simulink model "EV_PV_Charging"  (R2025a)
settings: Solver=ode3  StartTime=0.0  StopTime=1  RelTol=1e-3
PreLoadFcn:
  | %% Parameter file: OBC_4_data.m
  | 
  | %% Model Parameters
  | Ts_Power= 50e-9;        % SPS Model sample time (s)
  | Co=150e-6;              % Output filter (F)
  | Ron_FET=50e-3;          % FET resistance (ohms)
  | Ron_Diode=50e-3;        % FET resistance (ohms)
  | Vf=0.6;                 % Diode forward voltage (V)
  | %
  | %% PFC Data
  | Vnom_ac= 240;           % Nominal Ac voltage (V)
  | Fnom= 60;               % System frequency (Hz)
  | L_PFC= 600e-6;          % PFC Inductance (H)
  | RL_PFC= 20e-3;          % Inductance resistance (Ohm)
  | C_PFC= 2600e-6;         % Capacitance (F)
  | 
  | %% PFC Control System Parameters
  | Ts_Control= 10e-6;      % Control system time (s)
  | Fsw= 100e3;             % PWM Switching frequency (Hz)
  | DT_PFC=400e-9;
  | %
  | % Current Regulator (PR):
  | Kp_I= 0.06;             % Proportional gain
  | Kr_I= 2.5;              % Resonant gain
  | Zeta_I=0.2;             % Damping coefficient
  | Fr_I=Fnom*2;            % Resonant frequency (Hz)
  | %
  | % Voltage Regulator (PI):
  | Kp_V= 0.25;             % Proportional gain
  | Ki_V= 80;               % Integral gain
  | Limit_V= 100;           % Output limit
  | %
  | %% LLC Data
  | Vdc_in=400;             % DC input voltage (V)
  | Vo_nom=400;             % DC nominal output voltage (V)
  | Po_nom=7.2e3;           % Nominal output power (W)
  | Lr=25e-6;               % Transformer leakage inductance (Resonant inductance in Henry)
  | Lm=150e-6;              % Magnetization inductance (H)
  | Cr=75e-9;               % Resonant capacitor (F)
  | Np=10; Ns=12; N=Np/Ns;  % Transformer ratio
  | %
  | %% LLC Control System Parameters
  | DT_LLC=400e-9;
  | Ts_Control=10e-6;
  | % Voltage Regulator (PI):
  | Kp_LLC= 100/4;          % Proportional gain
  | Ki_LLC= 150e3;          % Integral gain
  | fs_LCC_min= 120e3;      % Minimum switching frequency (Hz)
  | fs_LCC_max= 300e3;      % Maximum switching frequency (Hz)
  | Vref_LCC_min= 275;      % Minimum voltage setpoint (V)
  | Vref_LCC_max= 450;      % Maximum voltage setpoint (V)
  | %
  | %%
  | % Resonant tank data
  | Ro=Vo_nom^2/Po_nom      % LLC output load (Ohm)
  | Rac=(8/pi^2)*N^2*Ro     % Equivalent pprimary AC resistance (Ohm)
  | Q=sqrt(Lr/Cr)/Rac       % Quality factor
  | fr=1/(2*pi*sqrt(Lr*Cr)) % Resonant frequency (Hz)
  | m=(Lr+Lm)/Lr            % Ratio of total primary reactance to resonant inductance (Lr)
  | %%
InitFcn:
  | %% Parameter file: OBC_4_data.m
  | 
  | %% Model Parameters
  | Ts_Power= 50e-9;        % SPS Model sample time (s)
  | Co=150e-6;              % Output filter (F)
  | Ron_FET=50e-3;          % FET resistance (ohms)
  | Ron_Diode=50e-3;        % FET resistance (ohms)
  | Vf=0.6;                 % Diode forward voltage (V)
  | %
  | %% PFC Data
  | Vnom_ac= 240;           % Nominal Ac voltage (V)
  | Fnom= 60;               % System frequency (Hz)
  | L_PFC= 600e-6;          % PFC Inductance (H)
  | RL_PFC= 20e-3;          % Inductance resistance (Ohm)
  | C_PFC= 2600e-6;         % Capacitance (F)
  | 
  | %% PFC Control System Parameters
  | Ts_Control= 10e-6;      % Control system time (s)
  | Fsw= 100e3;             % PWM Switching frequency (Hz)
  | DT_PFC=400e-9;
  | %
  | % Current Regulator (PR):
  | Kp_I= 0.06;             % Proportional gain
  | Kr_I= 2.5;              % Resonant gain
  | Zeta_I=0.2;             % Damping coefficient
  | Fr_I=Fnom*2;            % Resonant frequency (Hz)
  | %
  | % Voltage Regulator (PI):
  | Kp_V= 0.25;             % Proportional gain
  | Ki_V= 80;               % Integral gain
  | Limit_V= 100;           % Output limit
  | %
  | %% LLC Data
  | Vdc_in=400;             % DC input voltage (V)
  | Vo_nom=400;             % DC nominal output voltage (V)
  | Po_nom=7.2e3;           % Nominal output power (W)
  | Lr=25e-6;               % Transformer leakage inductance (Resonant inductance in Henry)
  | Lm=150e-6;              % Magnetization inductance (H)
  | Cr=75e-9;               % Resonant capacitor (F)
  | Np=10; Ns=12; N=Np/Ns;  % Transformer ratio
  | %
  | %% LLC Control System Parameters
  | DT_LLC=400e-9;
  | Ts_Control=10e-6;
  | % Voltage Regulator (PI):
  | Kp_LLC= 100/4;          % Proportional gain
  | Ki_LLC= 150e3;          % Integral gain
  | fs_LCC_min= 120e3;      % Minimum switching frequency (Hz)
  | fs_LCC_max= 300e3;      % Maximum switching frequency (Hz)
  | Vref_LCC_min= 275;      % Minimum voltage setpoint (V)
  | Vref_LCC_max= 450;      % Maximum voltage setpoint (V)
  | %
  | %%
  | % Resonant tank data
  | Ro=Vo_nom^2/Po_nom      % LLC output load (Ohm)
  | Rac=(8/pi^2)*N^2*Ro     % Equivalent pprimary AC resistance (Ohm)
  | Q=sqrt(Lr/Cr)/Rac       % Quality factor
  | fr=1/(2*pi*sqrt(Lr*Cr)) % Resonant frequency (Hz)
  | m=(Lr+Lm)/Lr            % Ratio of total primary reactance to resonant inductance (Lr)
  | %%
undefined symbols (not defined in the file or in its folder): D1, Delta, DiscIntNeverNeededParam
libraries: spsSeriesRLCBranchLib x11, spsDiodeLib x7, spsMeanLib x6, MyLibrary x6, spsCurrentMeasurementLib x5, spsVoltageMeasurementLib x5, spsFourierLib x4, spsThreePhaseTransformerTwoWindingsLib x3, spsOnDelayLib x3, spsDistributedParametersLineLib x2, spsThreePhaseParallelRLCLoadLib x2, spsPWMGeneratorDCDCLib x2
(part 3 of 4)

== system EV_PV_Charging/MPPT Controller using  'Incremental Conductance + Integral Regulator'  technique  ==
  V_PV : Inport
  I_PV : Inport  Port=2
  Add : Sum  Inputs=+-
  Deblock MPPT : Step  Time=0.4  SampleTime=0
  Duty Cycle : Constant  Value=Dinit
  MPPT : Subsystem
  PWM Generator (DC-DC) : spsPWMGeneratorDCDCLib/PWM Generator (DC-DC)  Fsw=fc  Ts=Ts_Power
  Saturation : Saturate  UpperLimit=1  LowerLimit=0
  Pulses : Outport  VectorParamsAs1DForOutWhenUnconnected=off
  tag scope: D=global
  wires:
  V_PV/1 -> MPPT/1(V_PV)
  I_PV/1 -> MPPT/2(I_PV)
  PWM Generator (DC-DC)/1 -> Pulses/1
  Deblock MPPT/1 -> MPPT/3(on/off)
  Saturation/1 -> PWM Generator (DC-DC)/1, [D]
  Add/1 -> Saturation/1  "D"
  MPPT/1(Delta_D) -> Add/2
  Duty Cycle/1 -> Add/1

== system EV_PV_Charging/Pmean ==
  Product : Product  RndMeth=Zero
  WkW : Gain  Gain=1/1000
  P : Outport  VectorParamsAs1DForOutWhenUnconnected=off
  V : Outport  Port=2  VectorParamsAs1DForOutWhenUnconnected=off
  wires:
  [Vmean_PV] -> Product/1, V/1
  Product/1 -> WkW/1
  [Imean_PV] -> Product/2
  WkW/1 -> P/1  "Pmean_PV (kW)"

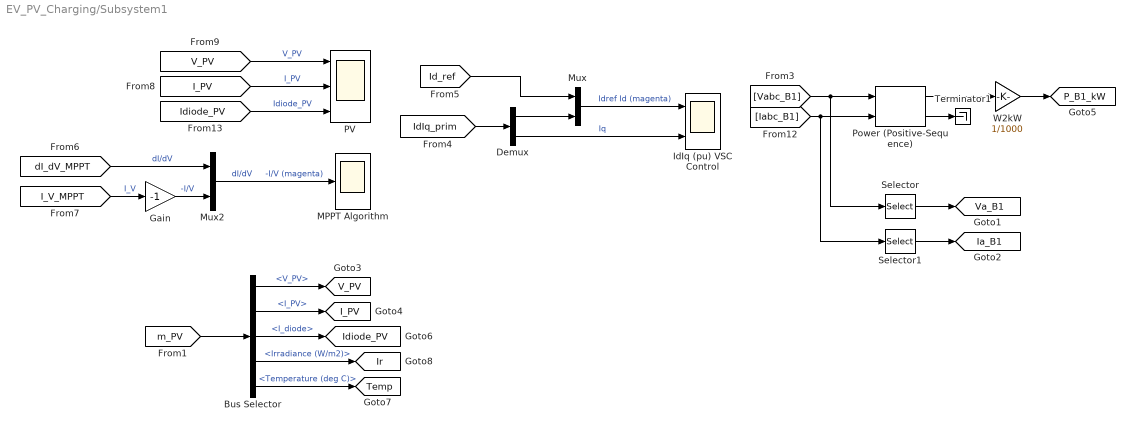
== system EV_PV_Charging/Subsystem1 ==
  Bus Selector : BusSelector  OutputSignals=V_PV,I_PV,I_diode,Irradiance (W/m2),Temperature (deg C)
  Demux : Demux  Outputs=2
  Gain : Gain  Gain=-1
  IdIq (pu) VSC Control : Scope  NumInputPorts=2
      settings: TimeSpan=2  ActiveDisplayYMinimum=-5  ActiveDisplayYMaximum=5  DataLoggingDecimation=100  DataLoggingSaveFormat=Array
  MPPT Algorithm : Scope
      settings: TimeSpan=2  DataLoggingDecimation=100  DataLoggingSaveFormat=Array
  Mux : Mux  Inputs=2
  Mux2 : Mux  Inputs=2
  PV : Scope  NumInputPorts=3
      settings: TimeSpan=2  ActiveDisplayYMinimum=-5  ActiveDisplayYMaximum=5  DataLoggingDecimation=100  DataLoggingSaveFormat=Array
  Power (Positive-Sequence) : spsPowerPositiveSequenceLib/Power (Positive-Sequence)  Freq=60  Vinit=[0, 0]  Iinit=[0, 0]  Ts=Ts_Control
  Selector : Selector  InputPortWidth=3  IndexOptions=Index vector (dialog)  Indices=[1]  OutputSizes=1
  Selector1 : Selector  InputPortWidth=3  IndexOptions=Index vector (dialog)  Indices=[1]  OutputSizes=1
  Terminator1 : Terminator
  W2kW : Gain  Gain=1/1000
  tag scope: I_PV=global, Ia_B1=global, Idiode_PV=global, Ir=global, P_B1_kW=global, Temp=global, V_PV=global, Va_B1=global
  wires:
  [Vabc_B1] -> Power (Positive-Sequence)/1, Selector/1
  [Iabc_B1] -> Power (Positive-Sequence)/2, Selector1/1
  Power (Positive-Sequence)/1 -> W2kW/1
  [I_V_MPPT] -> Gain/1  "I_V"
  [IdIq_prim] -> Demux/1
  [Id_ref] -> Mux/1
  Demux/1 -> Mux/2
  Mux/1 -> IdIq (pu) VSC Control/1  "Idref Id (magenta)"
  Demux/2 -> IdIq (pu) VSC Control/2  "Iq"
  Selector/1 -> [Va_B1]
  Selector1/1 -> [Ia_B1]
  [V_PV] -> PV/1  "V_PV"
  [I_PV] -> PV/2  "I_PV"
  [Idiode_PV] -> PV/3  "Idiode_PV"
  [dI_dV_MPPT] -> Mux2/1  "dI/dV"
  Gain/1 -> Mux2/2  "-I/V"
  Mux2/1 -> MPPT Algorithm/1  "dI/dV     -I/V (magenta)"
  W2kW/1 -> [P_B1_kW]
  [m_PV] -> Bus Selector/1
  Bus Selector/1 -> [V_PV]  "<V_PV>"
  Bus Selector/2 -> [I_PV]  "<I_PV>"
  Bus Selector/4 -> [Ir]  "<Irradiance (W/m2)>"
  Bus Selector/3 -> [Idiode_PV]  "<I_diode>"
  Bus Selector/5 -> [Temp]  "<Temperature (deg C)>"
  Power (Positive-Sequence)/2 -> Terminator1/1

== system EV_PV_Charging/Subsystem2 ==
  Mean : spsMeanLib/Mean  Freq=60  Vinit=0  Ts=Ts_Control
  Mux1 : Mux  Inputs=2
  Vm : Outport  VectorParamsAs1DForOutWhenUnconnected=off
  VrVm : Outport  Port=2  VectorParamsAs1DForOutWhenUnconnected=off
  wires:
  [Vdc_ref] -> Mux1/1  "Vdc ref"
  [Vdc] -> Mean/1  "Vdc"
  Mux1/1 -> VrVm/1
  Mean/1 -> Mux1/2, Vm/1

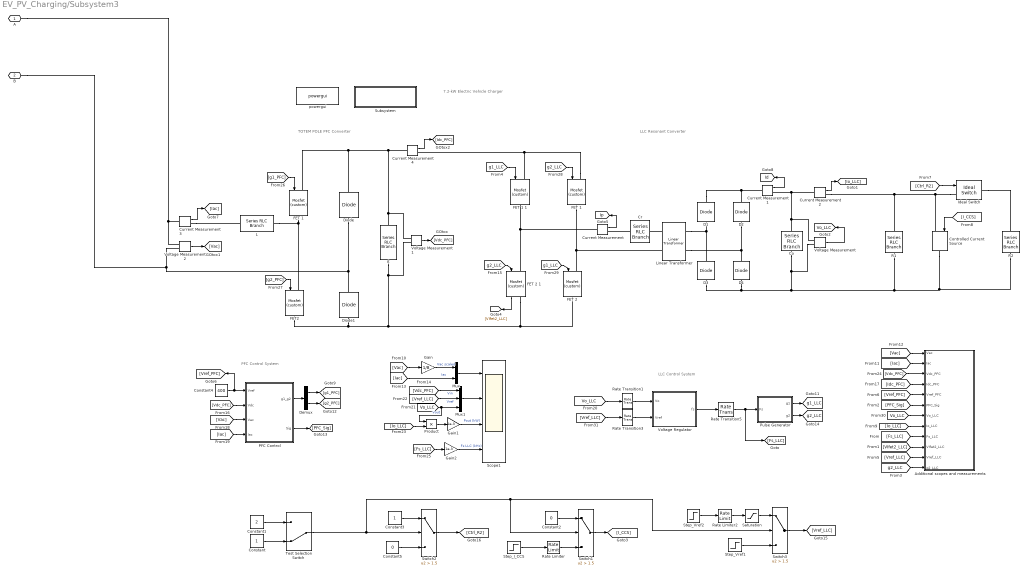
== system EV_PV_Charging/Subsystem3 ==
  note: TOTEM POLE PFC Converter
  note: 7.2-kW Electric Vehicle Charger
  note: LLC Control System
  note: PFC Control System
  note: LLC Resonant Converter
  Additional scopes and measurements : Subsystem
  C : spsSeriesRLCBranchLib/Series RLC Branch  LConnTagsString=__new0  RConnTagsString=__new0  BranchType=C  Resistance=1  Inductance=1e-3  SetiL0=off  InitialCurrent=0  Capacitance=C_PFC  Setx0=on  InitialVoltage=400  Measurements=None
  Co : spsSeriesRLCBranchLib/Series RLC Branch  LConnTagsString=__new0  RConnTagsString=__new0  BranchType=C  Resistance=1e-4  Inductance=200e-6  SetiL0=off  InitialCurrent=0  Capacitance=Co  Setx0=on  InitialVoltage=350  Measurements=None
  Constant : Constant
  Constant1 : Constant  Value=2
  Constant2 : Constant  Value=0
  Constant3 : Constant
  Constant4 : Constant  Value=400
  Constant5 : Constant  Value=0
  Controlled Current Source : spsControlledCurrentSourceLib/Controlled Current Source  Initialize=off  Source_Type=AC  Amplitude=0  Phase=0  Frequency=0  Measurements=None
  Cr : spsSeriesRLCBranchLib/Series RLC Branch  LConnTagsString=__new0  RConnTagsString=__new0  BranchType=C  Resistance=1e-4  Inductance=200e-6  SetiL0=off  InitialCurrent=0  Capacitance=Cr  Setx0=off  InitialVoltage=40  Measurements=None
  Current Measurement{,1..4} (5 alike) : spsCurrentMeasurementLib/Current Measurement  PhasorSimulation=off  OutputType=Complex  PSBequivalent=0
  D{1..4} (4 alike) : spsDiodeLib/Diode  Ron=Ron_Diode  Lon=0  Vf=Vf  IC=0  UseSnubber=off  Rs=1e6  Cs=inf  Measurements=off
  Demux : Demux  Outputs=2
  Diode : spsDiodeLib/Diode  Ron=Ron_Diode  Lon=0  Vf=Vf  IC=0  UseSnubber=0  Rs=1e6  Cs=inf  Measurements=off
  Diode1 : spsDiodeLib/Diode  Ron=Ron_Diode  Lon=0  Vf=Vf  IC=0  UseSnubber=0  Rs=1e6  Cs=inf  Measurements=off
  FET 1 : MyLibrary/Mosfet (custom)  Ron=Ron_FET  Lon=0  Rd=Ron_Diode  Vfd=Vf  IC=0  Rs=1e6  Cs=inf  Measurements=off
  "FET 1 " : MyLibrary/Mosfet (custom)  Ron=Ron_FET  Lon=0  Rd=Ron_Diode  Vfd=Vf  IC=0  Rs=1e6  Cs=inf  Measurements=off
  FET 1 1 : MyLibrary/Mosfet (custom)  Ron=Ron_FET  Lon=0  Rd=Ron_Diode  Vfd=Vf  IC=0  Rs=1e6  Cs=inf  Measurements=off
  "FET 2 " : MyLibrary/Mosfet (custom)  Ron=Ron_FET  Lon=0  Rd=Ron_Diode  Vfd=Vf  IC=0  Rs=1e6  Cs=inf  Measurements=off
  FET 2 1 : MyLibrary/Mosfet (custom)  Ron=Ron_FET  Lon=0  Rd=Ron_Diode  Vfd=Vf  IC=0  Rs=1e6  Cs=inf  Measurements=on
  FET2 : MyLibrary/Mosfet (custom)  Ron=Ron_FET  Lon=0  Rd=Ron_Diode  Vfd=Vf  IC=0  Rs=1e6  Cs=inf  Measurements=off
  Gain : Gain  Gain=1/8
  Gain1 : Gain  Gain=1e-3
  Gain2 : Gain  Gain=1e-3
  Ideal Switch : spsIdealSwitchLib/Ideal Switch  Ron=0.001  Lon=0  IC=0  Rs=1e6  Cs=inf  Measurements=off
  L : spsSeriesRLCBranchLib/Series RLC Branch  LConnTagsString=__new0  RConnTagsString=__new0  BranchType=RL  Resistance=RL_PFC  Inductance=L_PFC  SetiL0=off  InitialCurrent=0  Capacitance=1e-6  Setx0=off  InitialVoltage=0  Measurements=None
  Linear Transformer : spsLinearTransformerLib/Linear Transformer  UNITS=SI  NominalPower=[ 7000 100e3 ]  winding1="[Np   1e-2 Lr]"  winding2="[Ns  1e-2  1e-8 ]"  ThreeWindings=off  winding3=[3.15e+05 0.7938 0.084225]  RmLm=[1e4 Lm]  Measurements=None  DataType=on
  Mux : Mux  Inputs=2
  Mux1 : Mux  Inputs=3
  PFC Control : Subsystem
  Product : Product
  Pulse Generator : Subsystem
  R1 : spsSeriesRLCBranchLib/Series RLC Branch  LConnTagsString=__new0  RConnTagsString=__new0  BranchType=R  Resistance=Vo_nom^2/(0.01*Po_nom)  Inductance=200e-6  SetiL0=off  InitialCurrent=0  Capacitance=400e-6  Setx0=off  InitialVoltage=0  Measurements=None
  R2 : spsSeriesRLCBranchLib/Series RLC Branch  LConnTagsString=__new0  RConnTagsString=__new0  BranchType=R  Resistance=450^2/(Po_nom)  Inductance=200e-6  SetiL0=off  InitialCurrent=0  Capacitance=400e-6  Setx0=off  InitialVoltage=0  Measurements=None
  Rate Limiter : RateLimiter  RisingSlewLimit=200  FallingSlewLimit=-200  SampleTimeMode=inherited  InitialCondition=3
  Rate Limiter2 : RateLimiter  RisingSlewLimit=200*5  FallingSlewLimit=-200*5  SampleTimeMode=inherited  InitialCondition=250
  Rate Transition1 : RateTransition  OutPortSampleTime=Ts_Control
  Rate Transition3 : RateTransition  OutPortSampleTime=Ts_Control
  Rate Transition5 : RateTransition  InitialCondition=200e3  OutPortSampleTime=Ts_Power
  Saturation : Saturate  UpperLimit=Vref_LCC_max  LowerLimit=Vref_LCC_min
  Scope1 : Scope  NumInputPorts=4
      settings: ActiveDisplayYMinimum=-1863.73333  ActiveDisplayYMaximum=1350.80385  DataLoggingVariableName=ScopeData2
  Step_I_CCS : Step  Time=0.2  Before=3  After=18  SampleTime=Ts_Power
  Step_Vref1 : Step  Time=0.1  Before=350  After=400  SampleTime=Ts_Power
  Step_Vref2 : Step  Time=0.1  Before=250  After=450  SampleTime=Ts_Power
  Subsystem : Subsystem
      settings: OpenFcn=edit('OBC_v1_data');
      mask Display: disp('Double-click to open\n parameters file');
  Switch1 : Switch  Criteria=u2 > Threshold  Threshold=1.5  SaturateOnIntegerOverflow=off  InputSameDT=off
  Switch2 : Switch  Criteria=u2 > Threshold  Threshold=1.5  SaturateOnIntegerOverflow=off  InputSameDT=off
  Switch3 : Switch  Criteria=u2 > Threshold  Threshold=1.5  SaturateOnIntegerOverflow=off  InputSameDT=off
  Test Selection Switch : ManualSwitch  CurrentSetting=0
  Voltage Measurement : spsVoltageMeasurementLib/Voltage Measurement  PhasorSimulation=off  OutputType=Complex  PSBequivalent=0
  Voltage Measurement1 : spsVoltageMeasurementLib/Voltage Measurement  PhasorSimulation=off  OutputType=Complex  PSBequivalent=0
  Voltage Measurement2 : spsVoltageMeasurementLib/Voltage Measurement  PhasorSimulation=off  OutputType=Complex  PSBequivalent=0
  Voltage Regulator : Subsystem
  powergui : spspowerguiLib/powergui  Priority=1  SimulationMode=Discrete  SampleTime=Ts_Power  frequency=60  Iterations=50  frequencyindice=0  Pbase=100e6  ErrMax=1e-4  UnitsV=kV  UnitsW=MW  buscounter=0  FunctionMessages=off  echomessages=off  EnableUseOfTLC=off  CurrentSourceSwitches=off  DisableSnubberDevices=off  DisableRonSwitches=off  DisableVfSwitches=off  DisplayEquations=off  AutomaticDiscreteSolvers=off  SolverType=Tustin/Backward Euler (TBE)  Interpol=off  ExternalGateDelay=off  methode=off  Ts=100  x0status=blocks  SPID=on  SwTol=0  HookPort=off  NonlinearTolerance=1e-4  nMaxIteration=100  ContinueOnMaxIteration=off  RestoreLinks=warning  ResistiveCurrentMeasurement=off  Frange=[0:2:500]  Ylog=off  Xlog=on  ShowGrid=off  save=off  variable=ZData  structure=0  ZoomFFT=off  StartTime=0.0  cycles=1  DisplayStyle=1  fundamental=60  FreqAxis=off  MaxFrequency=1000  frequencyindicesteady=1  RmsSteady=1  display=off
  A : PMIOPort  Side=Left
  B : PMIOPort  Port=2  Side=Left
  tag scope: Id=global, Ip=global, Vo_LLC=global, g1_LLC=global, g2_LLC=global
  wires:
  Rate Transition5/1 -> [Fs_LLC], Pulse Generator/1(Fs)
  Voltage Measurement2/1 -> [Vac]
  Rate Transition1/1 -> Voltage Regulator/1(Vo)
  Voltage Regulator/1(fs) -> Rate Transition5/1
  Rate Transition3/1 -> Voltage Regulator/2(Vref)
  [Vdc_PFC] -> PFC Control/2(Vdc)
  Constant3/1 -> Switch2/1
  Rate Limiter2/1 -> Saturation/1
  Mux/1 -> Scope1/1
  Gain2/1 -> Scope1/4  "Fs LLC (kHz)"
  [Vdc_PFC] -> Additional scopes and measurements/3(Vdc_PFC)
  [Vref_LLC] -> Additional scopes and measurements/11(Vref_LLC)
  [Io_LLC] -> Additional scopes and measurements/8(Io_LLC)
  [g2_LLC] -> Additional scopes and measurements/12(g2_LLC)
  [Vo_LLC] -> Product/1, Mux1/3  "Vout"
  [Fs_LLC] -> Gain2/1
  Current Measurement3/1 -> [Iac]
  [g2_LLC] -> "FET 1 "/1
  [Idc_PFC] -> Additional scopes and measurements/4(Idc_PFC)
  [Vo_LLC] -> Additional scopes and measurements/7(Vo_LLC)
  [g2_PFC] -> FET2/1
  [Vac] -> Gain/1
  [Vref_PFC] -> Additional scopes and measurements/5(Vref_PFC)
  Voltage Measurement1/1 -> [Vdc_PFC]
  Constant1/1 -> Test Selection Switch/1
  [Vo_LLC] -> Rate Transition1/1
  Constant2/1 -> Switch1/1
  Gain/1 -> Mux/1  "Vac scaled"
  [Iac] -> PFC Control/4(Iac)
  Saturation/1 -> Switch3/1
  Pulse Generator/2(g2) -> [g2_LLC]
  [Iac] -> Mux/2  "Iac"
  Step_I_CCS/1 -> Rate Limiter/1
  [Vdc_PFC] -> Mux1/1  "Vin"
  PFC Control/2(Sig) -> [PFC_Sig]
  Voltage Measurement/1 -> [Vo_LLC]
  Rate Limiter/1 -> Switch1/3
  PFC Control/1(g1_g2) -> Demux/1
  Switch3/1 -> [Vref_LLC]
  [Iac] -> Additional scopes and measurements/2(Iac)
  [g1_PFC] -> FET 1/1
  [g1_LLC] -> FET 1 1/1
  FET 2 1/1 -> [VIfet2_LLC]
  Demux/1 -> [g1_PFC]
  Current Measurement/1 -> [Ip]
  Pulse Generator/1(g1) -> [g1_LLC]
  Test Selection Switch/1 -> Switch3/2, Switch1/2, Switch2/2
  [Fs_LLC] -> Additional scopes and measurements/9(Fs_LLC)
  [g1_LLC] -> "FET 2 "/1
  [Vac] -> PFC Control/3(Vac)
  Demux/2 -> [g2_PFC]
  Switch1/1 -> [I_CCS]
  Mux1/1 -> Scope1/2
  Constant/1 -> Test Selection Switch/2
  [Vref_LLC] -> Rate Transition3/1
  Step_Vref2/1 -> Rate Limiter2/1
  [Io_LLC] -> Product/2
  Current Measurement1/1 -> [Id]
  Product/1 -> Gain1/1
  [Vref_LLC] -> Mux1/2  "Vref"
  Current Measurement2/1 -> [Io_LLC]
  Current Measurement4/1 -> [Idc_PFC]
  [I_CCS] -> Controlled Current Source/1
  Constant4/1 -> [Vref_PFC], PFC Control/1(Vref)
  [Vac] -> Additional scopes and measurements/1(Vac)
  [VIfet2_LLC] -> Additional scopes and measurements/10(VIfet2_LLC)
  Constant5/1 -> Switch2/3
  Gain1/1 -> Scope1/3  "Pout (kW)"
  Switch2/1 -> [Ctrl_R2]
  [Ctrl_R2] -> Ideal Switch/1
  Step_Vref1/1 -> Switch3/3
  [g2_LLC] -> FET 2 1/1
  [PFC_Sig] -> Additional scopes and measurements/6(PFC_Sig)
  connections:
  D4/RConn1 -- D2/LConn1 -- Linear Transformer/RConn2
  Ideal Switch/LConn1 -- Current Measurement2/RConn1 -- R1/LConn1 -- Controlled Current Source/LConn1
  Voltage Measurement2/LConn2 -- B/RConn1 -- Diode/LConn1 -- Diode1/RConn1
  Voltage Measurement/LConn2 -- Co/RConn1 -- D4/LConn1 -- D3/LConn1 -- R2/RConn1 -- Controlled Current Source/RConn1 -- R1/RConn1
  D1/RConn1 -- D2/RConn1 -- Current Measurement1/LConn1
  Current Measurement1/RConn1 -- Current Measurement2/LConn1 -- Voltage Measurement/LConn1 -- Co/LConn1
  C/LConn1 -- Current Measurement4/LConn1 -- Diode/RConn1 -- FET 1/LConn1 -- Voltage Measurement1/LConn1
  FET 1 1/RConn1 -- FET 2 1/LConn1 -- Current Measurement/LConn1
  "FET 1 "/LConn1 -- FET 1 1/LConn1 -- Current Measurement4/RConn1
  Voltage Measurement2/LConn1 -- A/RConn1 -- Current Measurement3/LConn1
  "FET 2 "/RConn1 -- C/RConn1 -- Voltage Measurement1/LConn2 -- FET2/RConn1 -- Diode1/LConn1 -- FET 2 1/RConn1
  D3/RConn1 -- D1/LConn1 -- Linear Transformer/RConn1
  FET2/LConn1 -- L/RConn1 -- FET 1/RConn1
  "FET 1 "/RConn1 -- Linear Transformer/LConn2 -- "FET 2 "/LConn1
  Ideal Switch/RConn1 -- R2/LConn1
  Linear Transformer/LConn1 -- Cr/RConn1
  Current Measurement3/RConn1 -- L/LConn1
  Cr/LConn1 -- Current Measurement/RConn1

== system EV_PV_Charging/VSC Control ==
  note: VSC Main Controller
  Vabc_prim : Inport  PortDimensions=3
  Iabc_prim : Inport  Port=2  PortDimensions=3
  Vdc_mes : Inport  Port=3  PortDimensions=1
  Current Regulator : Subsystem
  Iq_ref : Constant  Value=0
  Mux : Mux  Inputs=2
  PLL & Measurements : Subsystem
  PWM Generator (3-Level) : spsPWMGenerator3LevelLib/PWM Generator (3-Level)  ModulatorType=Three-phase bridge (12 pulses)  ModulatorMode=Unsynchronized  nF=27  Fc=33*60  ModulatingSignals=off  m=0.8  Freq=60  Phase=0  Ts=Ts_Power
  Uabc_ref Generation max (m) = 1 : Subsystem
  Unit Delay : UnitDelay  SampleTime=Ts_Control  HasFrameUpgradeWarning=on
  VDC Regulator : Subsystem
  Vdc_ref1 : Constant  Value=Vdc_ref
  Pulses : Outport  VectorParamsAs1DForOutWhenUnconnected=off
  wires:
  VDC Regulator/1(Id_ref) -> Mux/1
  PLL & Measurements/1(wt) -> Uabc_ref Generation max (m) = 1/1(wt)
  Current Regulator/1(VdVq_conv) -> Uabc_ref Generation max (m) = 1/2(VdVq_conv)
  Iq_ref/1 -> Mux/2
  Mux/1 -> Current Regulator/3(IdIq_ref)
  PLL & Measurements/3(IdIq_prim) -> Current Regulator/2(IdIq_mes)
  PLL & Measurements/2(VdVq_prim) -> Current Regulator/1(VdVq_mes)
  Vdc_mes/1 -> VDC Regulator/1(Vdc_mes)
  Vabc_prim/1 -> PLL & Measurements/1(Vabc_prim)
  Iabc_prim/1 -> PLL & Measurements/2(Iabc_prim)
  Unit Delay/1 -> PWM Generator (3-Level)/1
  PWM Generator (3-Level)/1 -> Pulses/1
  Uabc_ref Generation max (m) = 1/1(Uabc_ref) -> Unit Delay/1
  Vdc_ref1/1 -> VDC Regulator/2(Vdc_ref)

== system EV_PV_Charging/info ==

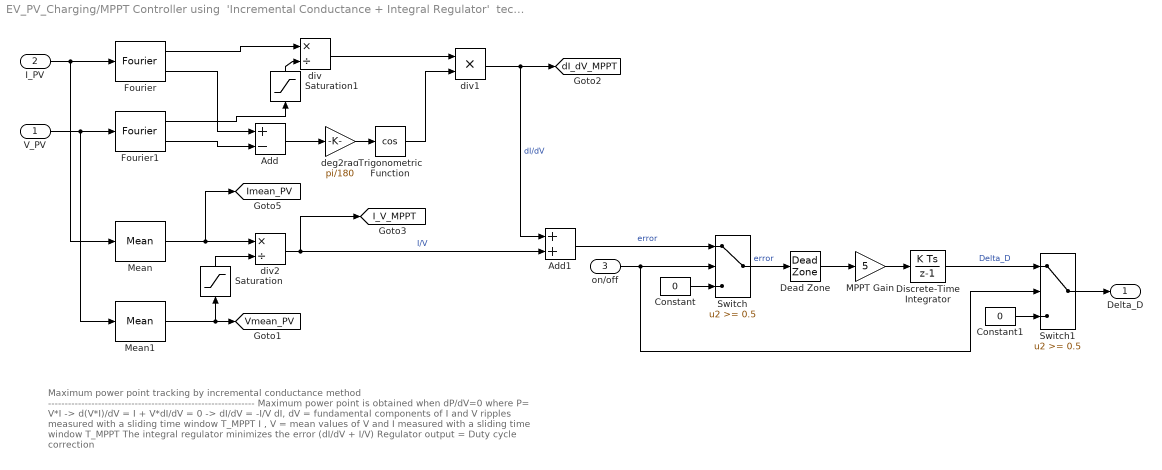
== system EV_PV_Charging/MPPT Controller using  'Incremental Conductance + Integral Regulator'  technique /MPPT ==
  note: Maximum power point tracking by incremental conductance method
      | --------------------------------------------------------------
      | Maximum power point is obtained when dP/dV=0  where P= V*I
      | -> d(V*I)/dV = I + V*dI/dV = 0
      | -> dI/dV = -I/V
      |
      | dI, dV  = fundamental components of I and V ripples measured with a sliding time window T_MPPT
      | I , V   = mean values of V and I measured with a sliding time window T_MPPT
      |
      | The integral regulator minimizes the error (dI/dV + I/V)
      | Regulator output = Duty cycle correction
  V_PV : Inport
  I_PV : Inport  Port=2
  on/off : Inport  Port=3
  Add : Sum  Inputs=+-
  Add1 : Sum
  Constant : Constant  Value=0
  Constant1 : Constant  Value=0
  Dead Zone : DeadZone  LowerValue=-0.05  UpperValue=0.05
  Discrete-Time Integrator : DiscreteIntegrator  SampleTime=Ts_Control  LimitOutput=on  UpperSaturationLimit=1  LowerSaturationLimit=-1  ICPrevOutput=DiscIntNeverNeededParam  ICPrevScaledInput=DiscIntNeverNeededParam
  Fourier : spsFourierLib/Fourier  Freq=1/T_MPPT  n=1  InInit=[0, 0]  Ts=Ts_Control
  Fourier1 : spsFourierLib/Fourier  Freq=1/T_MPPT  n=1  InInit=[0, 0]  Ts=Ts_Control
  MPPT Gain : Gain  Gain=5
  Mean : spsMeanLib/Mean  Freq=1/T_MPPT  Vinit=0  Ts=Ts_Control
  Mean1 : spsMeanLib/Mean  Freq=1/T_MPPT  Vinit=0  Ts=Ts_Control
  Saturation : Saturate  UpperLimit=inf  LowerLimit=eps
  Saturation1 : Saturate  UpperLimit=inf  LowerLimit=eps
  Switch : Switch  Threshold=0.5  SaturateOnIntegerOverflow=off  InputSameDT=off
  Switch1 : Switch  Threshold=0.5  SaturateOnIntegerOverflow=off  InputSameDT=off
  Trigonometric Function : Trigonometry  Operator=cos
  deg2rad : Gain  Gain=pi/180
  div : Product  Inputs=*/  RndMeth=Zero
  div1 : Product  Inputs=**  RndMeth=Zero
  div2 : Product  Inputs=*/  RndMeth=Zero
  Delta_D : Outport  VectorParamsAs1DForOutWhenUnconnected=off
  tag scope: I_V_MPPT=global, Imean_PV=global, Vmean_PV=global, dI_dV_MPPT=global
  wires:
  Dead Zone/1 -> MPPT Gain/1
  Switch/1 -> Dead Zone/1  "error"
  Saturation1/1 -> div/2
  Saturation/1 -> div2/2
  Switch1/1 -> Delta_D/1
  on/off/1 -> Switch/2, Switch1/2
  Constant1/1 -> Switch1/3
  Discrete-Time Integrator/1 -> Switch1/1  "Delta_D"
  Constant/1 -> Switch/3
  MPPT Gain/1 -> Discrete-Time Integrator/1
  Add1/1 -> Switch/1  "error"
  div2/1 -> Add1/2, [I_V_MPPT]  "I/V"
  Mean1/1 -> Saturation/1, [Vmean_PV]
  Mean/1 -> div2/1, [Imean_PV]
  div1/1 -> Add1/1, [dI_dV_MPPT]  "dI/dV"
  Trigonometric Function/1 -> div1/2
  div/1 -> div1/1
  deg2rad/1 -> Trigonometric Function/1
  Add/1 -> deg2rad/1
  Fourier1/1 -> Saturation1/1
  Fourier1/2 -> Add/2
  Fourier/2 -> Add/1
  V_PV/1 -> Mean1/1, Fourier1/1
  I_PV/1 -> Mean/1, Fourier/1
  Fourier/1 -> div/1

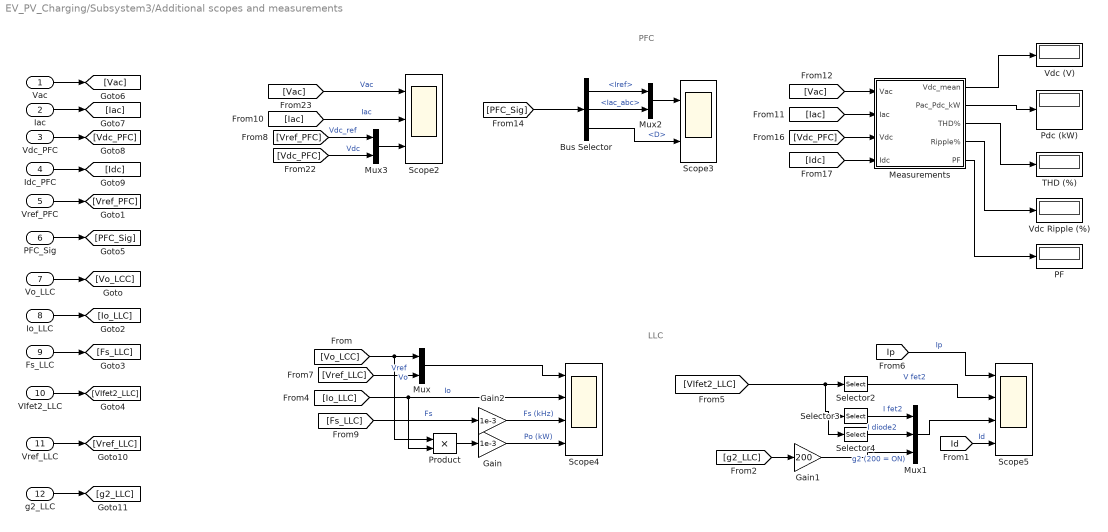
== system EV_PV_Charging/Subsystem3/Additional scopes and measurements ==
  note: PFC
  note: LLC
  Vac : Inport
  Iac : Inport  Port=2
  Vdc_PFC : Inport  Port=3
  Idc_PFC : Inport  Port=4
  Vref_PFC : Inport  Port=5
  PFC_Sig : Inport  Port=6
  Vo_LLC : Inport  Port=7
  Io_LLC : Inport  Port=8
  Fs_LLC : Inport  Port=9
  VIfet2_LLC : Inport  Port=10
  Vref_LLC : Inport  Port=11
  g2_LLC : Inport  Port=12
  Bus Selector : BusSelector  OutputSignals=Iref,Iac_abc,D
  Gain : Gain  Gain=1e-3
  Gain1 : Gain  Gain=200
  Gain2 : Gain  Gain=1e-3
  "Measurements " : Subsystem
  Mux : Mux  Inputs=2
  Mux1 : Mux  Inputs=3
  Mux2 : Mux  Inputs=2
  Mux3 : Mux  Inputs=2
  PF : Display
      settings: Format=bank  Decimation=100
  "Pdc (kW) " : Display
      settings: Format=bank  Decimation=100
  Product : Product
  Scope2 : Scope  NumInputPorts=3
      settings: ActiveDisplayYMinimum=-341.08729682378231  ActiveDisplayYMaximum=406.41106735822
  Scope3 : Scope  NumInputPorts=2
      settings: ActiveDisplayYMinimum=-9.06391  ActiveDisplayYMaximum=81.57518  DataLoggingVariableName=ScopeData2
  Scope4 : Scope  NumInputPorts=4
      settings: ActiveDisplayYMinimum=338.12925  ActiveDisplayYMaximum=441.6565  DataLoggingDecimation=10  DataLoggingVariableName=ScopeData2
  Scope5 : Scope  NumInputPorts=4
      settings: TimeSpan=0.00005  ActiveDisplayYMinimum=-148.13586  ActiveDisplayYMaximum=147.87237
  Selector2 : Selector  InputPortWidth=3  IndexOptions=Index vector (dialog)  Indices=2  OutputSizes=1
  Selector3 : Selector  InputPortWidth=3  IndexOptions=Index vector (dialog)  Indices=1  OutputSizes=1
  Selector4 : Selector  InputPortWidth=3  IndexOptions=Index vector (dialog)  Indices=3  OutputSizes=1
  "THD (%) " : Display
      settings: Format=bank  Decimation=100
  "Vdc (V) " : Display
      settings: Format=bank  Decimation=100
  Vdc Ripple (%) : Display
      settings: Format=bank  Decimation=100
  wires:
  Mux/1 -> Scope4/1
  [VIfet2_LLC] -> Selector4/1, Selector3/1, Selector2/1
  Selector2/1 -> Scope5/2  "V fet2"
  [Vac] -> Scope2/1  "Vac"
  Gain/1 -> Scope4/4  "Po (kW)"
  Mux1/1 -> Scope5/3
  [Ip] -> Scope5/1  "Ip"
  Selector4/1 -> Mux1/2  "I diode2"
  Bus Selector/3 -> Scope3/2  "<D>"
  Bus Selector/1 -> Mux2/1  "<Iref>"
  Bus Selector/2 -> Mux2/2  "<Iac_abc>"
  [Vo_LCC] -> Product/1, Mux/1  "Vo"
  [Vref_LLC] -> Mux/2  "Vref"
  Selector3/1 -> Mux1/1  "I fet2"
  "Measurements "/2(Pac_Pdc_kW) -> "Pdc (kW) "/1
  "Measurements "/4(Ripple%) -> Vdc Ripple (%)/1
  [Vdc_PFC] -> "Measurements "/3(Vdc)
  [Io_LLC] -> Product/2, Scope4/2  "Io"
  Mux2/1 -> Scope3/1
  Product/1 -> Gain/1
  [Vdc_PFC] -> Mux3/2  "Vdc"
  Mux3/1 -> Scope2/3
  [Id] -> Scope5/4  "Id"
  [PFC_Sig] -> Bus Selector/1
  [Idc] -> "Measurements "/4(Idc)
  [Vref_PFC] -> Mux3/1  "Vdc_ref"
  "Measurements "/5(PF) -> PF/1
  [Fs_LLC] -> Gain2/1  "Fs"
  "Measurements "/1(Vdc_mean) -> "Vdc (V) "/1
  [Iac] -> Scope2/2  "Iac"
  [Vac] -> "Measurements "/1(Vac)
  "Measurements "/3(THD%) -> "THD (%) "/1
  [Iac] -> "Measurements "/2(Iac)
  Vo_LLC/1 -> [Vo_LCC]
  Io_LLC/1 -> [Io_LLC]
  Fs_LLC/1 -> [Fs_LLC]
  VIfet2_LLC/1 -> [VIfet2_LLC]
  Vac/1 -> [Vac]
  Iac/1 -> [Iac]
  Vdc_PFC/1 -> [Vdc_PFC]
  Idc_PFC/1 -> [Idc]
  Vref_PFC/1 -> [Vref_PFC]
  PFC_Sig/1 -> [PFC_Sig]
  Vref_LLC/1 -> [Vref_LLC]
  g2_LLC/1 -> [g2_LLC]
  [g2_LLC] -> Gain1/1
  Gain1/1 -> Mux1/3  "g2 (200 = ON)"
  Gain2/1 -> Scope4/3  "Fs (kHz)"

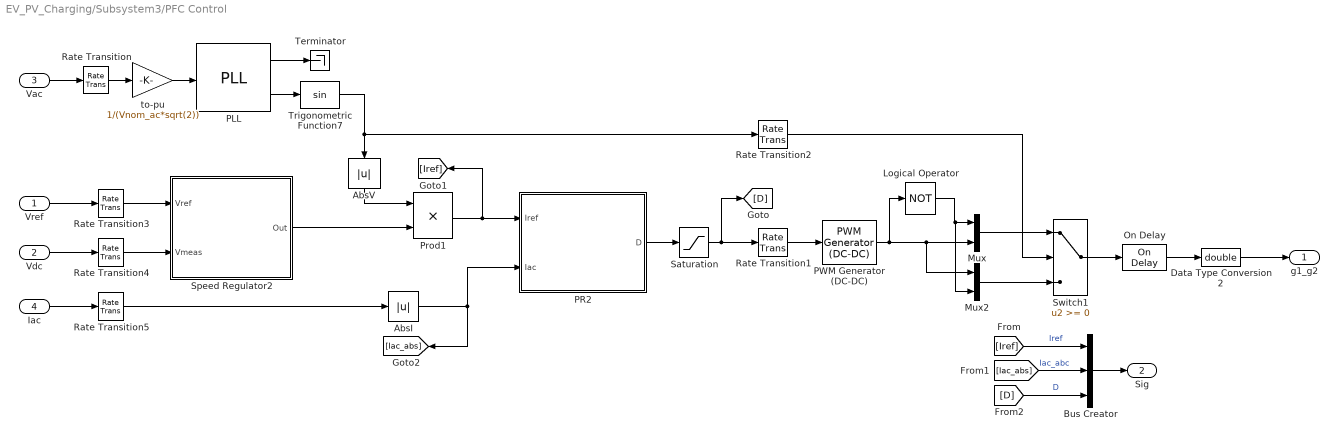
== system EV_PV_Charging/Subsystem3/PFC Control ==
  Vref : Inport
  Vdc : Inport  Port=2
  Vac : Inport  Port=3
  Iac : Inport  Port=4
  AbsI : Abs  SaturateOnIntegerOverflow=off
  AbsV : Abs  SaturateOnIntegerOverflow=off
  Bus Creator : BusCreator  Inputs=3
  Data Type Conversion2 : DataTypeConversion  OutDataTypeStr=double  SaturateOnIntegerOverflow=off  RndMeth=Floor
  Logical Operator : Logic  Operator=NOT  AllPortsSameDT=off  OutDataTypeStr=float('double')
  Mux : Mux  Inputs=2
  Mux2 : Mux  Inputs=2
  On Delay : spsOnDelayLib/On Delay  DelayType=On delay  delay=DT_PFC  ic=0  Ts=Ts_Power
  PLL : spsPLLLib/PLL  Fmin=0.9*Fnom  Par_Init=[0, Fnom]  ParK=[180, 3200, 1]  TcD=1e-4  MaxRateChangeFreq=12  FilterCutOffFreq=25  Ts=Ts_Control  AGC=on
  PR2 : Subsystem  mask(Current Regulator (Pr)){Kp=Kp_I, Kr=Kr_I, Fr=Fr_I}
      mask prompts: Kp "Proportional gain"; Kr "Resonant gain"; Fr "Resonant frequency (Hz)"
      mask help: This block implements a currentregulator using a PR controller.
      mask Display: disp('Current Regulator\n PR');
  PWM Generator (DC-DC) : spsPWMGeneratorDCDCLib/PWM Generator (DC-DC)  Fsw=Fsw  Ts=Ts_Power
  Prod1 : Product
  Rate Transition{,3..5} (4 alike) : RateTransition  OutPortSampleTime=Ts_Control
  Rate Transition1 : RateTransition  OutPortSampleTime=Ts_Power
  Rate Transition2 : RateTransition  OutPortSampleTime=Ts_Power
  Saturation : Saturate  UpperLimit=1  LowerLimit=0
  Speed Regulator2 : Subsystem  DialogController=POWERSYS.PowerSysDialog  mask(Voltage Regulator){Kp=Kp_V, Ki=Ki_V, Limit_wreg=Limit_V, Init=0, Ts=Ts_Control}
      mask prompts: Kp "Proportional gain (Kp):"; Ki "Integral gain (Ki):"; Limit_wreg "Output limits"; Init "Output initial value:"; Ts "Sample time:"
      mask help: This block implements a voltage regulator using an ant-windup PI controller.
      mask Display: disp('Voltage\nRegulator');
  Switch1 : Switch  SaturateOnIntegerOverflow=off  InputSameDT=off
  Terminator : Terminator
  Trigonometric Function7 : Trigonometry
  to-pu : Gain  Gain=1/(Vnom_ac*sqrt(2))
  g1_g2 : Outport  PortDimensions=2
  Sig : Outport  Port=2
  wires:
  Vdc/1 -> Rate Transition4/1
  Speed Regulator2/1(Out) -> Prod1/2
  Vac/1 -> Rate Transition/1
  AbsV/1 -> Prod1/1
  Vref/1 -> Rate Transition3/1
  Prod1/1 -> PR2/1(Iref), [Iref]
  AbsI/1 -> PR2/2(Iac), [Iac_abs]
  Saturation/1 -> [D], Rate Transition1/1
  Mux/1 -> Switch1/1
  Mux2/1 -> Switch1/3
  Rate Transition1/1 -> PWM Generator (DC-DC)/1
  Bus Creator/1 -> Sig/1
  [Iref] -> Bus Creator/1  "Iref"
  [Iac_abs] -> Bus Creator/2  "Iac_abc"
  [D] -> Bus Creator/3  "D"
  Switch1/1 -> On Delay/1
  PWM Generator (DC-DC)/1 -> Logical Operator/1, Mux2/1, Mux/2
  to-pu/1 -> PLL/1
  PLL/2 -> Trigonometric Function7/1
  Trigonometric Function7/1 -> AbsV/1, Rate Transition2/1
  PLL/1 -> Terminator/1
  PR2/1(D) -> Saturation/1
  Logical Operator/1 -> Mux2/2, Mux/1
  Rate Transition2/1 -> Switch1/2
  Rate Transition/1 -> to-pu/1
  Rate Transition3/1 -> Speed Regulator2/1(Vref)
  Rate Transition4/1 -> Speed Regulator2/2(Vmeas)
  Rate Transition5/1 -> AbsI/1
  Iac/1 -> Rate Transition5/1
  On Delay/1 -> Data Type Conversion2/1
  Data Type Conversion2/1 -> g1_g2/1

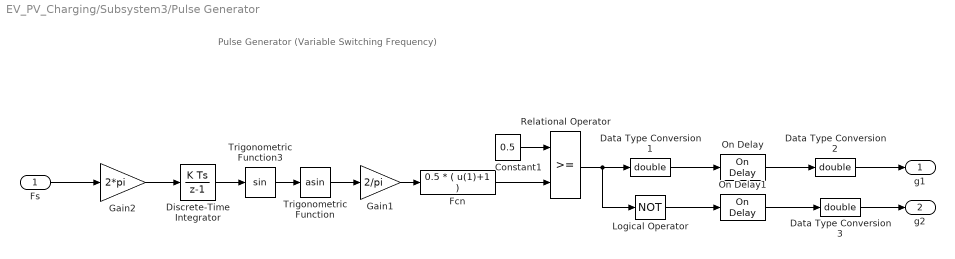
== system EV_PV_Charging/Subsystem3/Pulse Generator ==
  note: Pulse Generator
      | (Variable Switching Frequency)
  Fs : Inport
  Constant1 : Constant  Value=0.5
  Data Type Conversion1 : DataTypeConversion  OutDataTypeStr=double  SaturateOnIntegerOverflow=off  RndMeth=Floor
  Data Type Conversion2 : DataTypeConversion  OutDataTypeStr=double  SaturateOnIntegerOverflow=off  RndMeth=Floor
  Data Type Conversion3 : DataTypeConversion  OutDataTypeStr=double  SaturateOnIntegerOverflow=off  RndMeth=Floor
  Discrete-Time Integrator : DiscreteIntegrator  SampleTime=Ts_Power  ICPrevOutput=DiscIntNeverNeededParam  ICPrevScaledInput=DiscIntNeverNeededParam
  Fcn : Fcn  Expr=0.5 * ( u(1)+1 )
  Gain1 : Gain  Gain=2/pi  SaturateOnIntegerOverflow=on  OutDataTypeStr=Inherit: Same as input  ParamDataTypeStr=Inherit: Same as input
  Gain2 : Gain  Gain=2*pi  SaturateOnIntegerOverflow=on  OutDataTypeStr=Inherit: Same as input  ParamDataTypeStr=Inherit: Same as input
  Logical Operator : Logic  Operator=NOT  AllPortsSameDT=off  OutDataTypeStr=float('double')
  On Delay : spsOnDelayLib/On Delay  DelayType=On delay  delay=DT_LLC  ic=0  Ts=Ts_Power
  On Delay1 : spsOnDelayLib/On Delay  DelayType=On delay  delay=DT_LLC  ic=0  Ts=Ts_Power
  Relational Operator : RelationalOperator  OutDataTypeStr=boolean  InputSameDT=off
  Trigonometric Function : Trigonometry  Operator=asin
  Trigonometric Function3 : Trigonometry
  g1 : Outport  VectorParamsAs1DForOutWhenUnconnected=off
  g2 : Outport  Port=2  VectorParamsAs1DForOutWhenUnconnected=off
  wires:
  On Delay1/1 -> Data Type Conversion3/1
  On Delay/1 -> Data Type Conversion2/1
  Fs/1 -> Gain2/1
  Gain2/1 -> Discrete-Time Integrator/1
  Data Type Conversion1/1 -> On Delay/1
  Logical Operator/1 -> On Delay1/1
  Fcn/1 -> Relational Operator/2
  Relational Operator/1 -> Logical Operator/1, Data Type Conversion1/1
  Constant1/1 -> Relational Operator/1
  Discrete-Time Integrator/1 -> Trigonometric Function3/1
  Trigonometric Function/1 -> Gain1/1
  Gain1/1 -> Fcn/1
  Trigonometric Function3/1 -> Trigonometric Function/1
  Data Type Conversion2/1 -> g1/1
  Data Type Conversion3/1 -> g2/1

== system EV_PV_Charging/Subsystem3/Subsystem ==

== system EV_PV_Charging/Subsystem3/Voltage Regulator ==
  Vo : Inport
  Vref : Inport  Port=2
  Discrete-Time Integrator2 : DiscreteIntegrator  InitialCondition=fs_LCC_min  SampleTime=Ts_Control  LimitOutput=on  UpperSaturationLimit=fs_LCC_max  LowerSaturationLimit=fs_LCC_min  ICPrevOutput=DiscIntNeverNeededParam  ICPrevScaledInput=DiscIntNeverNeededParam
  Gain1 : Gain  Gain=Kp_LLC  SaturateOnIntegerOverflow=on  OutDataTypeStr=Inherit: Same as input  ParamDataTypeStr=Inherit: Same as input
  Gain4 : Gain  Gain=Ki_LLC  SaturateOnIntegerOverflow=on  OutDataTypeStr=Inherit: Same as input  ParamDataTypeStr=Inherit: Same as input
  Saturation1 : Saturate  UpperLimit=fs_LCC_max  LowerLimit=fs_LCC_min
  Sum1 : Sum  Inputs=|+-  InputSameDT=on  SaturateOnIntegerOverflow=on  OutDataTypeStr=Inherit: Same as first input
  Sum2 : Sum  InputSameDT=on  SaturateOnIntegerOverflow=on  OutDataTypeStr=Inherit: Same as first input
  fs : Outport  VectorParamsAs1DForOutWhenUnconnected=off
  wires:
  Saturation1/1 -> fs/1
  Gain1/1 -> Sum2/1
  Sum2/1 -> Saturation1/1
  Discrete-Time Integrator2/1 -> Sum2/2
  Gain4/1 -> Discrete-Time Integrator2/1
  Sum1/1 -> Gain4/1, Gain1/1
  Vo/1 -> Sum1/1
  Vref/1 -> Sum1/2

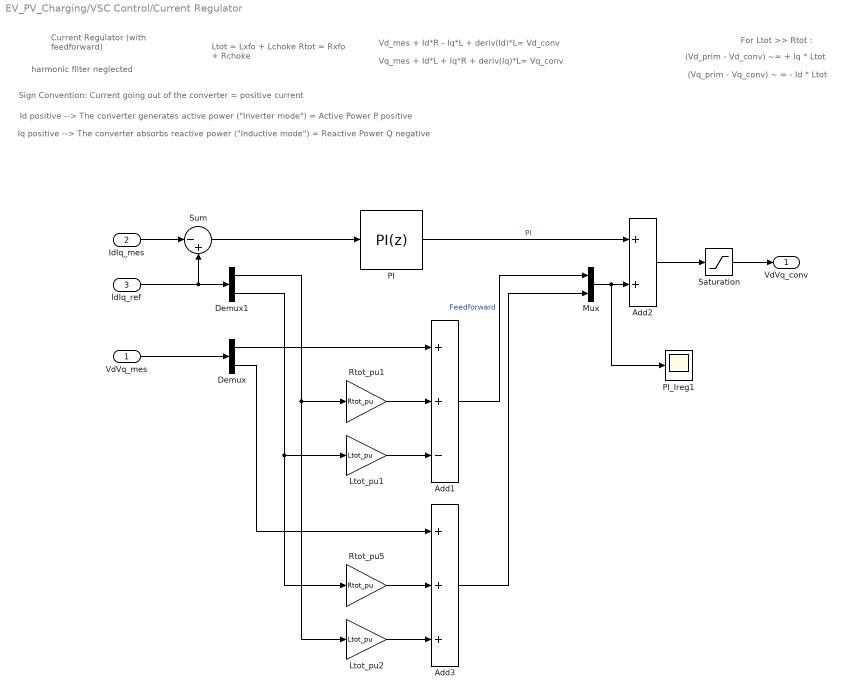
== system EV_PV_Charging/VSC Control/Current Regulator ==
  note: harmonic filter neglected
  note: Vd_mes + Id*R - Iq*L + deriv(Id)*L= Vd_conv
  note: Vq_mes + Id*L + Iq*R + deriv(Iq)*L= Vq_conv
  note: Current Regulator
      | (with feedforward)
  note: Sign Convention: Current going out of the converter = positive current
  note: Iq positive --> The converter absorbs reactive power ("Inductive mode") = Reactive Power Q negative
  note: Id positive --> The converter generates active power ("Inverter mode") = Active Power P positive
  note: Ltot = Lxfo + Lchoke
      | Rtot = Rxfo + Rchoke
  note: (Vd_prim - Vd_conv) ~= + Iq * Ltot
  note: (Vq_prim - Vq_conv) ~ = - Id * Ltot
  note: For Ltot >> Rtot :
  VdVq_mes : Inport  PortDimensions=2
  IdIq_mes : Inport  Port=2  PortDimensions=2
  IdIq_ref : Inport  Port=3  PortDimensions=2
  Add1 : Sum  Inputs=++-
  Add2 : Sum
  Add3 : Sum  Inputs=+++
  Demux : Demux  Outputs=2
  Demux1 : Demux  Outputs=2
  Ltot_pu1 : Gain  Gain=Ltot_pu  SaturateOnIntegerOverflow=on  OutDataTypeStr=Inherit: Same as input  ParamDataTypeStr=Inherit: Same as input
  Ltot_pu2 : Gain  Gain=Ltot_pu  SaturateOnIntegerOverflow=on  OutDataTypeStr=Inherit: Same as input  ParamDataTypeStr=Inherit: Same as input
  Mux : Mux  Inputs=2
  PI : slpidlib/PID Controller  Controller=PI  Form=Parallel  TimeDomain=Discrete-time  UseExternalTs=off  SampleTime=Ts  IntegratorMethod=Forward Euler  FilterMethod=Forward Euler  ControllerParametersSource=internal  P=Kp_Ireg  I=Ki_Ireg  UseKiTs=off  D=0  UseExternalDerivativeSource=off  N=100  UseFilter=on  TunerSelectOption=Transfer Function Based (PID Tuner App)  InitialConditionSource=internal  InitialConditionForIntegrator=0  InitialConditionForFilter=0  DifferentiatorICPrevScaledInput=0  ExternalReset=none  TrackingMode=off  Kt=1  LimitOutput=on  SatLimitsSource=internal  UpperSaturationLimit=2  LowerSaturationLimit=-2  LinearizeAsGain=off  AntiWindupMode=none  Kb=1  LimitIntegrator=off  UpperIntegratorSaturationLimit=inf  LowerIntegratorSaturationLimit=-inf  POutMin=[]  POutMax=[]  IOutMin=[]  IOutMax=[]  DOutMin=[]  DOutMax=[]  NOutMin=[]  NOutMax=[]  SumOutMin=[]  SumOutMax=[]  SaturationOutMin=[]  SaturationOutMax=[]  PParamMin=[]  PParamMax=[]  IParamMin=[]  IParamMax=[]  DParamMin=[]  DParamMax=[]  NParamMin=[]  NParamMax=[]  KbParamMin=[]  KbParamMax=[]  KtParamMin=[]  KtParamMax=[]  KbOutMin=[]  KbOutMax=[]  KtOutMin=[]  KtOutMax=[]  IntegratorOutMin=[]  IntegratorOutMax=[]  FilterOutMin=[]  FilterOutMax=[]  SumI1OutMin=[]  SumI1OutMax=[]  SumI2OutMin=[]  SumI2OutMax=[]  SumI3OutMin=[]  SumI3OutMax=[]  SumI4OutMin=[]  SumI4OutMax=[]  SumDOutMin=[]  SumDOutMax=[]  DifferentiatorOutMin=[]  DifferentiatorOutMax=[]  FilterDiffOutCoefMin=[]  FilterDiffOutCoefMax=[]  ReciprocalOutMin=[]  ReciprocalOutMax=[]  SumDenOutMin=[]  SumDenOutMax=[]  SumNumOutMin=[]  SumNumOutMax=[]  DivideOutMin=[]  DivideOutMax=[]  UdiffTsProdOutMin=[]  UdiffTsProdOutMax=[]  NTsProdOutMin=[]  NTsProdOutMax=[]  UintegralTsProdOutMin=[]  UintegralTsProdOutMax=[]  UngainTsProdOutMin=[]  UngainTsProdOutMax=[]  ClampingZeroOutDataTypeStr=Inherit: Inherit via back propagation  ClampingZeroOutMin=[]  ClampingZeroOutMax=[]  FilterDenConstantOutDataTypeStr=Inherit: Inherit via back propagation  FilterDenConstantOutMin=[]  FilterDenConstantOutMax=[]  PCopyOutDataTypeStr=Inherit: Inherit via back propagation  PCopyOutMin=[]  PCopyOutMax=[]  NCopyOutDataTypeStr=Inherit: Inherit via back propagation  NCopyOutMin=[]  NCopyOutMax=[]  IntegratorContinuousStateAttributes=''  IntegratorStateMustResolveToSignalObject=off  IntegratorRTWStateStorageClass=Auto  FilterContinuousStateAttributes=''  FilterStateMustResolveToSignalObject=off  FilterRTWStateStorageClass=Auto  ParallelPVariant=InternalParameters  IdealPVariant=Disabled  IVariant=InternalParameters  DVariant=Disabled  IntegratorVariant=Discrete  SatVariant=Enabled  AWVariant=Passthrough  PCopyVariant=Disabled  TRVariant=Disabled  FdbkBlocksVariant=Forward  IdealPFdbkVariant=Disabled  SatFdbkVariant=Disabled  DerivativeFilterVariant=Disabled  NVariant=Disabled  NCopyVariant=Disabled_SignalSpec  FilterICVariant=Disabled  IntegratorICVariant=InternalICs  ExternalResetVariant=Disabled  TRSumVariant=Passthrough  SumFdbkVariant=Disabled  SumVariant=Sum_PI  TsampFilterVariant=InternalTs  TsampNgainVariant=Passthrough  TsampIntegralVariant=Disabled_SignalSpec  ExternalSaturationOutDataTypeStr=Inherit: Same as second input  DerivativeSourceVariant=Disabled  PreIntVariant=InternalPreInt
  PI_Ireg1 : Scope
      settings: DataLoggingSaveFormat=Array
  Rtot_pu1 : Gain  Gain=Rtot_pu  SaturateOnIntegerOverflow=on  OutDataTypeStr=Inherit: Same as input  ParamDataTypeStr=Inherit: Same as input
  Rtot_pu5 : Gain  Gain=Rtot_pu  SaturateOnIntegerOverflow=on  OutDataTypeStr=Inherit: Same as input  ParamDataTypeStr=Inherit: Same as input
  Saturation : Saturate  UpperLimit=2  LowerLimit=-2
  Sum : Sum  Inputs=|-+
  VdVq_conv : Outport  VectorParamsAs1DForOutWhenUnconnected=off
  wires:
  Mux/1 -> PI_Ireg1/1, Add2/2
  PI/1 -> Add2/1  "PI"
  Sum/1 -> PI/1
  IdIq_ref/1 -> Sum/2, Demux1/1
  IdIq_mes/1 -> Sum/1
  Add2/1 -> Saturation/1
  Saturation/1 -> VdVq_conv/1
  VdVq_mes/1 -> Demux/1
  Demux/1 -> Add1/1
  Rtot_pu1/1 -> Add1/2
  Demux1/1 -> Rtot_pu1/1, Ltot_pu2/1
  Ltot_pu1/1 -> Add1/3
  Demux1/2 -> Ltot_pu1/1, Rtot_pu5/1
  Rtot_pu5/1 -> Add3/2
  Ltot_pu2/1 -> Add3/3
  Add1/1 -> Mux/1  "Feedforward"
  Demux/2 -> Add3/1
  Add3/1 -> Mux/2

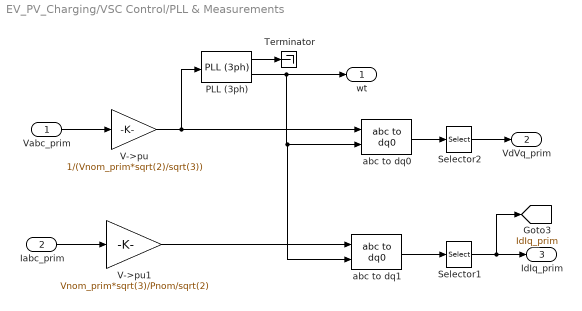
== system EV_PV_Charging/VSC Control/PLL & Measurements ==
  Vabc_prim : Inport
  Iabc_prim : Inport  Port=2
  PLL (3ph) : spsPLL3phLib/PLL (3ph)  Fmin=45  Par_Init="[-0.57  Fnom]"  ParK=[180, 3200, 1]  TcD=1e-4  MaxRateChangeFreq=12  FilterCutOffFreq=25  Ts=Ts  AGC=on
  Selector1 : Selector  InputPortWidth=3  IndexOptions=Index vector (dialog)  Indices=[1 2]  OutputSizes=1
  Selector2 : Selector  InputPortWidth=3  IndexOptions=Index vector (dialog)  Indices=[1 2]  OutputSizes=1
  Terminator : Terminator
  V->pu : Gain  Gain=1/(Vnom_prim*sqrt(2)/sqrt(3))  SaturateOnIntegerOverflow=on  OutDataTypeStr=Inherit: Same as input  ParamDataTypeStr=Inherit: Same as input
  V->pu1 : Gain  Gain=Vnom_prim*sqrt(3)/Pnom/sqrt(2)  SaturateOnIntegerOverflow=on  OutDataTypeStr=Inherit: Same as input  ParamDataTypeStr=Inherit: Same as input
  abc to dq0 : spsabctodq0Lib/abc to dq0  Alignment=90 degrees behind phase A axis
  abc to dq1 : spsabctodq0Lib/abc to dq0  Alignment=90 degrees behind phase A axis
  wt : Outport  VectorParamsAs1DForOutWhenUnconnected=off
  VdVq_prim : Outport  Port=2  VectorParamsAs1DForOutWhenUnconnected=off
  IdIq_prim : Outport  Port=3  VectorParamsAs1DForOutWhenUnconnected=off
  tag scope: IdIq_prim=global
  wires:
  V->pu1/1 -> abc to dq1/1
  V->pu/1 -> PLL (3ph)/1, abc to dq0/1
  abc to dq1/1 -> Selector1/1
  Vabc_prim/1 -> V->pu/1
  Iabc_prim/1 -> V->pu1/1
  abc to dq0/1 -> Selector2/1
  Selector2/1 -> VdVq_prim/1
  Selector1/1 -> [IdIq_prim], IdIq_prim/1
  PLL (3ph)/2 -> wt/1, abc to dq1/2, abc to dq0/2
  PLL (3ph)/1 -> Terminator/1

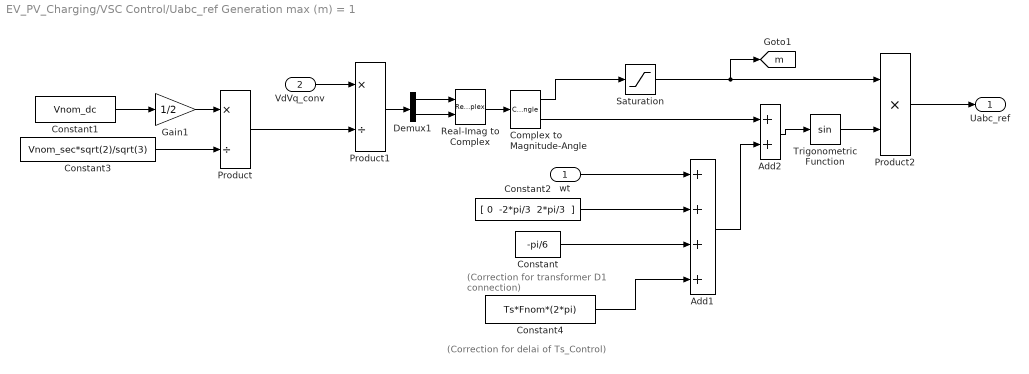
== system EV_PV_Charging/VSC Control/Uabc_ref Generation max (m) = 1 ==
  note: (Correction for transformer
      |  D1 connection)
  note: (Correction for delai of Ts_Control)
  wt : Inport
  VdVq_conv : Inport  Port=2
  Add1 : Sum  Inputs=++++
  Add2 : Sum
  Complex to Magnitude-Angle : ComplexToMagnitudeAngle
  Constant : Constant  Value=-pi/6
  Constant1 : Constant  Value=Vnom_dc
  Constant2 : Constant  Value="[ 0  -2*pi/3  2*pi/3  ]"
  Constant3 : Constant  Value=Vnom_sec*sqrt(2)/sqrt(3)
  Constant4 : Constant  Value=Ts*Fnom*(2*pi)
  Demux1 : Demux  Outputs=2
  Gain1 : Gain  Gain=1/2
  Product : Product  Inputs=*/  RndMeth=Zero
  Product1 : Product  Inputs=*/  RndMeth=Zero
  Product2 : Product  Inputs=**  RndMeth=Zero
  Real-Imag to Complex : RealImagToComplex
  Saturation : Saturate  UpperLimit=1  LowerLimit=0
  Trigonometric Function : Trigonometry
  Uabc_ref : Outport  VectorParamsAs1DForOutWhenUnconnected=off
  tag scope: m=global
  wires:
  Complex to Magnitude-Angle/1 -> Saturation/1
  Constant1/1 -> Gain1/1
  VdVq_conv/1 -> Product1/1
  Product1/1 -> Demux1/1
  Gain1/1 -> Product/1
  Real-Imag to Complex/1 -> Complex to Magnitude-Angle/1
  Demux1/1 -> Real-Imag to Complex/1
  Demux1/2 -> Real-Imag to Complex/2
  Constant2/1 -> Add1/2
  Constant/1 -> Add1/3
  Constant3/1 -> Product/2
  Product/1 -> Product1/2
  Complex to Magnitude-Angle/2 -> Add2/1
  Add1/1 -> Add2/2
  Add2/1 -> Trigonometric Function/1
  Saturation/1 -> [m], Product2/1
  Trigonometric Function/1 -> Product2/2
  Product2/1 -> Uabc_ref/1
  wt/1 -> Add1/1
  Constant4/1 -> Add1/4

== system EV_PV_Charging/VSC Control/VDC Regulator ==
  Vdc_mes : Inport  PortDimensions=1
  Vdc_ref : Inport  Port=2  PortDimensions=1
  PI : slpidlib/PID Controller  Controller=PI  Form=Parallel  TimeDomain=Discrete-time  UseExternalTs=off  SampleTime=Ts  IntegratorMethod=Trapezoidal  FilterMethod=Forward Euler  ControllerParametersSource=internal  P=Kp_VDCreg  I=Ki_VDCreg  UseKiTs=off  D=0  UseExternalDerivativeSource=off  N=100  UseFilter=on  TunerSelectOption=Transfer Function Based (PID Tuner App)  InitialConditionSource=internal  InitialConditionForIntegrator=0  InitialConditionForFilter=0  DifferentiatorICPrevScaledInput=0  ExternalReset=none  TrackingMode=off  Kt=1  LimitOutput=on  SatLimitsSource=internal  UpperSaturationLimit=1.5  LowerSaturationLimit=-1.5  LinearizeAsGain=off  AntiWindupMode=none  Kb=1  LimitIntegrator=off  UpperIntegratorSaturationLimit=inf  LowerIntegratorSaturationLimit=-inf  POutMin=[]  POutMax=[]  IOutMin=[]  IOutMax=[]  DOutMin=[]  DOutMax=[]  NOutMin=[]  NOutMax=[]  SumOutMin=[]  SumOutMax=[]  SaturationOutMin=[]  SaturationOutMax=[]  PParamMin=[]  PParamMax=[]  IParamMin=[]  IParamMax=[]  DParamMin=[]  DParamMax=[]  NParamMin=[]  NParamMax=[]  KbParamMin=[]  KbParamMax=[]  KtParamMin=[]  KtParamMax=[]  KbOutMin=[]  KbOutMax=[]  KtOutMin=[]  KtOutMax=[]  IntegratorOutMin=[]  IntegratorOutMax=[]  FilterOutMin=[]  FilterOutMax=[]  SumI1OutMin=[]  SumI1OutMax=[]  SumI2OutMin=[]  SumI2OutMax=[]  SumI3OutMin=[]  SumI3OutMax=[]  SumI4OutMin=[]  SumI4OutMax=[]  SumDOutMin=[]  SumDOutMax=[]  DifferentiatorOutMin=[]  DifferentiatorOutMax=[]  FilterDiffOutCoefMin=[]  FilterDiffOutCoefMax=[]  ReciprocalOutMin=[]  ReciprocalOutMax=[]  SumDenOutMin=[]  SumDenOutMax=[]  SumNumOutMin=[]  SumNumOutMax=[]  DivideOutMin=[]  DivideOutMax=[]  UdiffTsProdOutMin=[]  UdiffTsProdOutMax=[]  NTsProdOutMin=[]  NTsProdOutMax=[]  UintegralTsProdOutMin=[]  UintegralTsProdOutMax=[]  UngainTsProdOutMin=[]  UngainTsProdOutMax=[]  ClampingZeroOutDataTypeStr=Inherit: Inherit via back propagation  ClampingZeroOutMin=[]  ClampingZeroOutMax=[]  FilterDenConstantOutDataTypeStr=Inherit: Inherit via back propagation  FilterDenConstantOutMin=[]  FilterDenConstantOutMax=[]  PCopyOutDataTypeStr=Inherit: Inherit via back propagation  PCopyOutMin=[]  PCopyOutMax=[]  NCopyOutDataTypeStr=Inherit: Inherit via back propagation  NCopyOutMin=[]  NCopyOutMax=[]  IntegratorContinuousStateAttributes=''  IntegratorStateMustResolveToSignalObject=off  IntegratorRTWStateStorageClass=Auto  FilterContinuousStateAttributes=''  FilterStateMustResolveToSignalObject=off  FilterRTWStateStorageClass=Auto  ParallelPVariant=InternalParameters  IdealPVariant=Disabled  IVariant=InternalParameters  DVariant=Disabled  IntegratorVariant=Discrete  SatVariant=Enabled  AWVariant=Passthrough  PCopyVariant=Disabled  TRVariant=Disabled  FdbkBlocksVariant=Forward  IdealPFdbkVariant=Disabled  SatFdbkVariant=Disabled  DerivativeFilterVariant=Disabled  NVariant=Disabled  NCopyVariant=Disabled_SignalSpec  FilterICVariant=Disabled  IntegratorICVariant=InternalICs  ExternalResetVariant=Disabled  TRSumVariant=Passthrough  SumFdbkVariant=Disabled  SumVariant=Sum_PI  TsampFilterVariant=InternalTs  TsampNgainVariant=Passthrough  TsampIntegralVariant=Disabled_SignalSpec  ExternalSaturationOutDataTypeStr=Inherit: Same as second input  DerivativeSourceVariant=Disabled  PreIntVariant=InternalPreInt
  Rtot_pu3 : Gain  Gain=1/Vnom_dc  SaturateOnIntegerOverflow=on  OutDataTypeStr=Inherit: Same as input  ParamDataTypeStr=Inherit: Same as input
  Sum : Sum  Inputs=|+-
  Id_ref : Outport  SampleTime=Ts  InitialOutput=0  VectorParamsAs1DForOutWhenUnconnected=off
  tag scope: Id_ref=global, Vdc_ref=global
  wires:
  Sum/1 -> Rtot_pu3/1
  Vdc_mes/1 -> Sum/1
  Vdc_ref/1 -> Sum/2, [Vdc_ref]
  Rtot_pu3/1 -> PI/1
  PI/1 -> [Id_ref], Id_ref/1

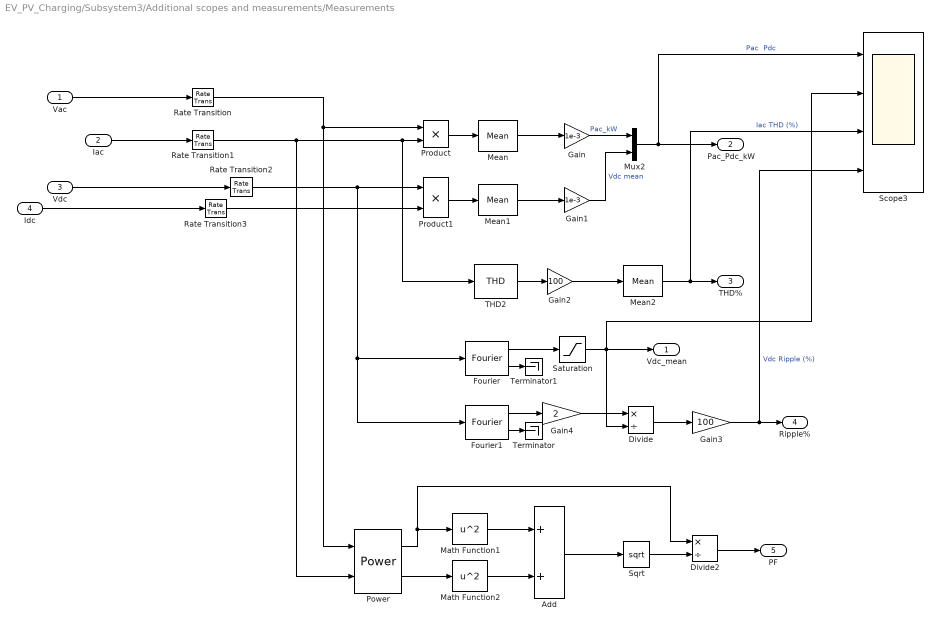
== system EV_PV_Charging/Subsystem3/Additional scopes and measurements/Measurements  ==
  Vac : Inport
  Iac : Inport  Port=2
  Vdc : Inport  Port=3
  Idc : Inport  Port=4
  Add : Sum
  Divide : Product  Inputs=*/
  Divide2 : Product  Inputs=*/
  Fourier : spsFourierLib/Fourier  Freq=Fnom  n=0  InInit=[0, 0]  Ts=Ts_Control
  Fourier1 : spsFourierLib/Fourier  Freq=Fnom  n=2  InInit=[0, 0]  Ts=Ts_Control
  Gain : Gain  Gain=1e-3
  Gain1 : Gain  Gain=1e-3
  Gain2 : Gain  Gain=100
  Gain3 : Gain  Gain=100
  Gain4 : Gain  Gain=2
  Math Function1 : Math  Operator=square
  Math Function2 : Math  Operator=square
  Mean : spsMeanLib/Mean  Freq=Fnom  Vinit=0  Ts=Ts_Control
  Mean1 : spsMeanLib/Mean  Freq=Fnom  Vinit=0  Ts=Ts_Control
  Mean2 : spsMeanLib/Mean  Freq=Fnom  Vinit=0  Ts=Ts_Control
  Mux2 : Mux  Inputs=2
  Power : spsPowerLib/Power  Freq=Fnom  Vinit=[1, 0]  Iinit=[1, 0]  Ts=Ts_Control
  Product : Product
  Product1 : Product
  Rate Transition{,1..3} (4 alike) : RateTransition  OutPortSampleTime=Ts_Control
  Saturation : Saturate  UpperLimit=inf  LowerLimit=eps
  Scope3 : Scope  NumInputPorts=4
      settings: ActiveDisplayYMinimum=-1.32447  ActiveDisplayYMaximum=11.92024
  Sqrt : Sqrt
  THD2 : spsTHDLib/THD  Freq=Fnom  Ts=Ts_Control
  Terminator : Terminator
  Terminator1 : Terminator
  Vdc_mean : Outport
  Pac_Pdc_kW : Outport  Port=2
  THD% : Outport  Port=3
  Ripple% : Outport  Port=4
  PF : Outport  Port=5
  wires:
  Gain1/1 -> Mux2/2  "Vdc mean"
  Product1/1 -> Mean1/1
  Mean/1 -> Gain/1
  Product/1 -> Mean/1
  Gain/1 -> Mux2/1  "Pac_kW"
  THD2/1 -> Gain2/1
  Mean1/1 -> Gain1/1
  Iac/1 -> Rate Transition1/1
  Mux2/1 -> Scope3/1, Pac_Pdc_kW/1  "Pac  Pdc"
  Gain2/1 -> Mean2/1
  Mean2/1 -> Scope3/3, THD%/1  "Iac THD (%)"
  Fourier/2 -> Terminator1/1
  Fourier/1 -> Saturation/1
  Saturation/1 -> Scope3/2, Vdc_mean/1, Divide/2
  Divide/1 -> Gain3/1
  Fourier1/1 -> Gain4/1
  Gain4/1 -> Divide/1
  Fourier1/2 -> Terminator/1
  Gain3/1 -> Scope3/4, Ripple%/1  "Vdc Ripple (%)"
  Power/1 -> Math Function1/1, Divide2/1
  Power/2 -> Math Function2/1
  Math Function1/1 -> Add/1
  Math Function2/1 -> Add/2
  Add/1 -> Sqrt/1
  Sqrt/1 -> Divide2/2
  Divide2/1 -> PF/1
  Rate Transition1/1 -> Power/2, THD2/1, Product/2
  Vdc/1 -> Rate Transition2/1
  Idc/1 -> Rate Transition3/1
  Rate Transition/1 -> Power/1, Product/1
  Vac/1 -> Rate Transition/1
  Rate Transition2/1 -> Product1/1, Fourier/1, Fourier1/1
  Rate Transition3/1 -> Product1/2

== system EV_PV_Charging/Subsystem3/PFC Control/PR2 ==
  Iref : Inport
  Iac : Inport  Port=2
  Gain : Gain  Gain=Kp
  Gain1 : Gain  Gain=Kr
  Second-Order Filter1 : spsSecondOrderFilterLib/Second-Order Filter  FilterType=Bandpass  Fo=Fr  Zeta=Zeta_I  Ts=Ts_Control  Initialize=off  Vac_Init="[0,  0,  60]"  Vdc_Init=0  PlotResponse=off  FreqRange=[0, 1000, 0.2]
  Sum1 : Sum  Inputs=|+-
  Sum2 : Sum  Inputs=|++
  D : Outport
  wires:
  Gain1/1 -> Second-Order Filter1/1
  Sum2/1 -> D/1
  Gain/1 -> Sum2/1
  Iac/1 -> Sum1/2
  Iref/1 -> Sum1/1
  Sum1/1 -> Gain1/1, Gain/1
  Second-Order Filter1/1 -> Sum2/2
